simulink model "FFM_Punch"  (R2017a)
settings: Solver=ode3  StartTime=0.0  StopTime=timesteps  FixedStep=data.SIM.Ts  RelTol=1e-3  EnableMultiTasking=on
values from neighbouring files (symbols this model uses):
  data =     [dakota_config.mat]
  downshift_map = data.TCU.upshift.veh_spd_default    [Simulation_results.m]
  upshift_map = data.TCU.upshift.veh_spd_default    [Simulation_results.m]
undefined symbols (not defined in the file or in its folder): air_density, Cd, DiscIntNeverNeededParam, fr_crankshaft, fr_speed_values, g, i_FD, ICE, Low_Ratio, M_Eng_Max, M_Eng_Max_Max, M_Eng_Max_Rpm, mt2m_f, mu_Roll_C0, mu_Roll_C1, mu_Roll_C2, Mv, n_Idle_Eng, Overdrive_Ratio, Re, S_eff_drag, Ts
(part 1 of 15)
settings Model: Creator=37sr  LastModifiedBy=DOM
settings SolverCC: MaxConsecutiveMinStep=Ts
settings DataIOCC: SaveFormat=Array  InspectSignalLogs=on
settings OptimizationCC: LifeSpan=inf
settings DebuggingCC: InheritedTsInSrcMsg=none  ParameterPrecisionLossMsg=none  SFUnexpectedBacktrackingDiag=warning  SFNoUnconditionalDefaultTransitionDiag=warning  SFExecutionAtInitializationDiag=none
settings HardwareCC: ProdBitPerPointer=32  ProdBitPerSizeT=32  ProdBitPerPtrDiffT=32  ProdLargestAtomicFloat=None  ProdIntDivRoundTo=Undefined  ProdEndianess=Unspecified  ProdWordSize=32  ProdHWDeviceType=32-bit Generic
settings ModelReferenceCC: PropagateSignalLabelsOutOfModel=off
settings GRTTargetCC: TargetLangStandard=C89/C90 (ANSI)  GeneratePreprocessorConditionals=Disable all
settings ConfigComp: CovMetricSettings=dw  CovHtmlReporting=on  CovSaveCumulativeToWorkspaceVar=on  CovSaveSingleToWorkspaceVar=on  CovExternalEMLEnable=off
settings ConfigurationSet: Description=SimMechanics 2G

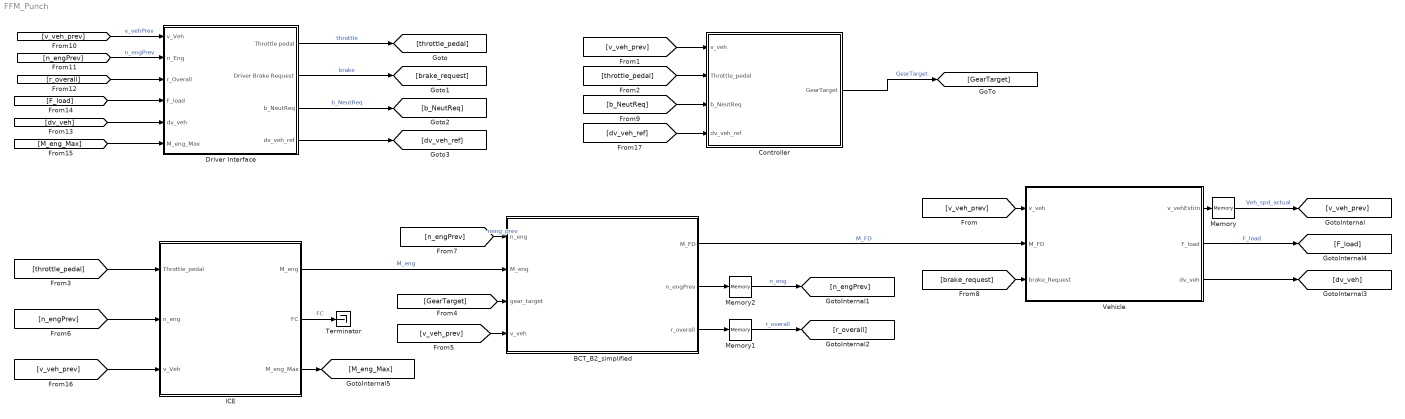
== system FFM_Punch ==
  BCT_B2_simplified : Subsystem
      mask Display:
      | port_label('input',1,'n_eng')
      | port_label('input',2,'M_eng')
      | port_label('input',4,'v_veh')
      | port_label('input',3,'GearTarget')
      | port_label('output',1,'M_FD')
  Controller : Subsystem  Tag=Controls_Lib  Description=SubSystem
      settings: RTWSystemCode=Inline
  Driver Interface : Subsystem
  ICE : Subsystem  SystemSampleTime=Ts/10
      mask Display:
      | port_label('input',1,'Throttle pedal')
      | port_label('input',2,'Engine speed')
      | port_label('output',1,'M_eng')
      | port_label('output',2,'FC')
      | color('blue')
  Memory : Memory  InheritSampleTime=on  LinearizeMemory=on  LinearizeAsDelay=on
  Memory1 : Memory
  Memory2 : Memory  X0=data.ENG.idle_speed
  Terminator : Terminator
      settings: Tag=Controls_Lib  Description=Terminator
  Vehicle : Subsystem  DialogController=PMDialogs.PMDefaultMaskDlg
      mask Display:
      | port_label('input', 1, 'v_veh');
      | port_label('input', 2, 'M_FD');
      | port_label('output', 1, 'v_veh');
  wires:
  Vehicle/1(v_vehEstim) -> Memory/1
  Memory/1 -> [v_veh_prev]  "Veh_spd_actual"
  [v_veh_prev] -> Vehicle/1(v_veh)
  [v_veh_prev] -> Controller/1(v_veh)
  ICE/1(M_eng) -> BCT_B2_simplified/2(M_eng)  "M_eng"
  BCT_B2_simplified/1(M_FD) -> Vehicle/2(M_FD)  "M_FD"
  [throttle_pedal] -> Controller/2(Throttle_pedal)
  [throttle_pedal] -> ICE/1(Throttle_pedal)
  Controller/1(GearTarget) -> [GearTarget]  "GearTarget"
  [v_veh_prev] -> BCT_B2_simplified/4(v_veh)
  BCT_B2_simplified/2(n_engPrev) -> Memory2/1
  [n_engPrev] -> ICE/2(n_eng)
  [n_engPrev] -> BCT_B2_simplified/1(n_eng)  "neng_prev"
  Driver Interface/1(Throttle pedal) -> [throttle_pedal]  "throttle"
  Driver Interface/2(Driver Brake Request) -> [brake_request]  "brake"
  [brake_request] -> Vehicle/3(brake_Request)
  Driver Interface/3(b_NeutReq) -> [b_NeutReq]  "b_NeutReq"
  [b_NeutReq] -> Controller/3(b_NeutReq)
  BCT_B2_simplified/3(r_overall) -> Memory1/1
  ICE/2(FC) -> Terminator/1  "FC"
  [v_veh_prev] -> Driver Interface/1(v_Veh)  "v_vehPrev"
  [n_engPrev] -> Driver Interface/2(n_Eng)  "n_engPrev"
  [r_overall] -> Driver Interface/3(r_Overall)
  Memory2/1 -> [n_engPrev]  "n_eng"
  Memory1/1 -> [r_overall]  "r_overall"
  [GearTarget] -> BCT_B2_simplified/3(gear_target)
  Vehicle/2(F_load) -> [F_load]  "F_load"
  [F_load] -> Driver Interface/4(F_load)
  [v_veh_prev] -> ICE/3(v_Veh)
  Vehicle/3(dv_veh) -> [dv_veh]
  [dv_veh] -> Driver Interface/5(dv_veh)
  ICE/3(M_eng_Max) -> [M_eng_Max]
  [M_eng_Max] -> Driver Interface/6(M_eng_Max)
  Driver Interface/4(dv_veh_ref) -> [dv_veh_ref]
  [dv_veh_ref] -> Controller/4(dv_veh_ref)

== system FFM_Punch/BCT_B2_simplified ==
  n_eng : Inport
  M_eng : Inport  Port=2
  gear_target : Inport  Port=3
  v_veh : Inport  Port=4
  Efficiency_Simplified_Model : Subsystem
  GearBox : Subsystem
      mask Display: image(imread('BCT1_GearCluster.jpg'));
  M_FD : Outport
  n_engPrev : Outport  Port=2
  r_overall : Outport  Port=3
  wires:
  n_eng/1 -> [n_eng]
  M_eng/1 -> [M_inpMeas]
  [M_inpMeas] -> Efficiency_Simplified_Model/2(M_inpMeas)
  [n_eng] -> Efficiency_Simplified_Model/3(n_Eng)
  gear_target/1 -> [gear_target]
  [gear_target] -> Efficiency_Simplified_Model/1(gear_target)
  [gear_target] -> GearBox/1(gear_target)
  Efficiency_Simplified_Model/1(M_inpLoss) -> GearBox/2(M_inpLoss)
  GearBox/1(M_FD) -> M_FD/1
  v_veh/1 -> [v_veh]
  GearBox/2(n_engPrev) -> n_engPrev/1
  [v_veh] -> GearBox/3(v_veh)
  GearBox/3(r_overall) -> r_overall/1

== system FFM_Punch/Controller ==
  v_veh : Inport  Tag=Controls_Lib  Description=Inp  Interpolate=off
  Throttle_pedal : Inport  Port=2
  b_NeutReq : Inport  Port=3
  dv_veh_ref : Inport  Tag=Controls_Lib  Description=Inp  Port=4  Interpolate=off
  F02_03_03_03_Shift_Laws_Determination : Subsystem
  F02_03_03_05_Raw_Gear_Target_Auto_Mode : Subsystem
  Scope : Scope  NumInputPorts=2
  Scope1 : Scope
  Scope2 : Scope
  UnitDelay : UnitDelay  Tag=Controls_Lib  Description=UnitDelay  InitialCondition=X0  SampleTime=SampleTime  mask(Unit delay){X0=0, InputProcessing=Elements as channels (sample based), SampleTime=-1, StateIdentifier=, StateMustResolveToSignalObject=off, RTWStateStorageClass=Auto, RTWStateStorageTypeQualifier=}
      mask prompts: X0 "Initial conditions:"; InputProcessing "Input processing:"; SampleTime "Sample time (-1 for inherited):"; StateIdentifier "State name:"; StateMustResolveToSignalObject "State name must resolve to Simulink signal object"; RTWStateStorageClass "Code generation storage class:"; RTWStateStorageTypeQualifier "Code generation storage type qualifier:"
      mask help: Delays input signal by one sample period
      settings: AttributesFormatString=Init_con=%<X0>
      mask Help: web([fileparts(which('Lib_discrete')) filesep 'hlp' filesep 'lib_UnitDelay.html'], '-helpbrowser')
      mask TypeOptions X0: X0
      mask TypeOptions InputProcessing: InputProcessing
      mask TypeOptions SampleTime: SampleTime
      mask TypeOptions StateIdentifier: StateIdentifier
      mask TypeOptions StateMustResolveToSignalObject: StateMustResolveToSignalObject
      mask TypeOptions RTWStateStorageClass: RTWStateStorageClass
      mask TypeOptions RTWStateStorageTypeQualifier: RTWStateStorageTypeQualifier
  GearTarget : Outport  Tag=Controls_Lib  Description=Out  InitialOutput=0
  wires:
  Throttle_pedal/1 -> F02_03_03_03_Shift_Laws_Determination/1(Throttle_pedal)
  F02_03_03_03_Shift_Laws_Determination/1(ts_v_vectThdAutoModDown) -> Scope1/1, [ts_v_vectThdAutoModDown]
  F02_03_03_03_Shift_Laws_Determination/2(ts_v_vectThdAutoModUp) -> Scope2/1, [ts_v_vectThdAutoModUp]
  [ts_v_vectThdAutoModDown] -> F02_03_03_05_Raw_Gear_Target_Auto_Mode/1(ts_v_vectThdAutoModDown)
  [ts_v_vectThdAutoModUp] -> F02_03_03_05_Raw_Gear_Target_Auto_Mode/2(ts_v_vectThdAutoModUp)
  [ts_z_gearTgtFwd] -> F02_03_03_05_Raw_Gear_Target_Auto_Mode/3(ts_z_gearTgtFwd)
  v_veh/1 -> Scope/2, F02_03_03_05_Raw_Gear_Target_Auto_Mode/4(vehest_v_frntWhl)
  F02_03_03_05_Raw_Gear_Target_Auto_Mode/1(ts_z_autoGearTgtRaw) -> UnitDelay/1, GearTarget/1
  UnitDelay/1 -> [ts_z_gearTgtFwd]
  b_NeutReq/1 -> F02_03_03_05_Raw_Gear_Target_Auto_Mode/5(b_NeutReq)
  [dv_veh_ref] -> F02_03_03_05_Raw_Gear_Target_Auto_Mode/6(dv_veh_ref)
  dv_veh_ref/1 -> Scope/1, [dv_veh_ref]

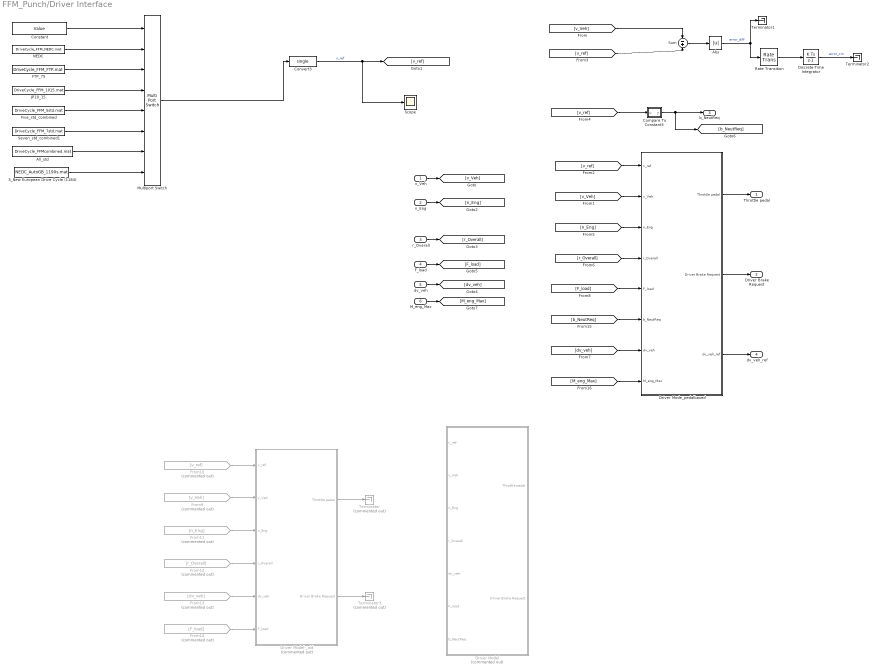
== system FFM_Punch/Driver Interface ==
  v_Veh : Inport
  n_Eng : Inport  Port=2
  r_Overall : Inport  Port=3
  F_load : Inport  Port=4
  dv_veh : Inport  Port=5
  M_eng_Max : Inport  Port=6
  3_New European Drive Cycle (1184) : FromFile  FileName=NEDC_AutoGB_1190s.mat  SampleTime=data.SIM.Ts
  Abs : Abs
  All_std : FromFile  FileName=DriveCycle_FFMcombined.mat  SampleTime=0
  Compare To Constant3 : Subsystem  mask(Compare To Constant){relop=<, const=0.5, OutDataTypeStr=boolean, ZeroCross=off}
      mask prompts: relop "Simulink:masks:Operator_MP"; const "Simulink:masks:ConstantValue_MP"; OutDataTypeStr "Simulink:masks:OutputDataType_MP"; ZeroCross "Simulink:masks:EnableZerocrossingDetection_MP"
      mask help: Simulink:masks:CompareToConstant_MD
      mask init:
      | blkName = gcb;
      | 
      | if strcmp(get_param(gcbh,'OutDataTypeStr'),'boolean')
      | 	setValue = 'boolean';
      | else
      | 	setValue = 'fixdt(0, 8)';
      | end
      | 
      | set_param([blkName,'/Compare'],'relop',relop, ...
      | 	'OutDataTypeStr', setValue, 'ZeroCross', ZeroCross);
      | 
      | str = [relop,' C']; %default
      | 
      | const_str = get_param(blkName, 'const');
      | const_val = str2num(const_str);
      | 
      | if isempty(const_val) %#ok<ST2NM>
      |     %Expression/Variable
      |     str = [relop, ' ', strtrim(const_str)];
      | else
      |     if length(const_val) == 1 
      |         if Simulink.data.isSupportedEnumClass(class(const_val))
      |             % Special Handling for Enumerations
      |             if Simulink.data.getEnumTypeInfo(class(const_val), 'AddClassNameToEnumNames')
      |                 str = [relop, ' ', strtrim(const_str)];
      |             else
      |                 str = [relop, ' ', char(const_val)];
      |             end
      |         elseif(isfloat(const_val) || isinteger(const_val)) 
      |                 str = [relop, ' ', num2str(const_val)];
      |         end
      |     end
      | end
      mask TypeOptions relop: == | ~= | < | <= | >= | >
      mask TypeOptions OutDataTypeStr: Simulink:masks:uint8 | Simulink:masks:boolean
      mask Callback ZeroCross: sl('zeroCrossEnable', gcbh);
      mask Display: disp(str)
  Constant : Constant  Tag=Controls_Lib  Description=constant  Value=Value  OutMin=OutMin  OutMax=OutMax  OutDataTypeStr=Inherit: Inherit via back propagation  SampleTime=SampleTime  FramePeriod=FramePeriod  mask(Constant){Value=data.SIM.drivecycle, VectorParams1D=on, SampleTime=-1, FramePeriod=inf, OutMin=[], OutMax=[], OutDataTypeStr=Inherit: Inherit via back propagation, LockScale=off}
      mask prompts: Value "Simulink:blkprm_prompts:ConstConstValue"; VectorParams1D "Simulink:blkprm_prompts:AllSrcsVector1D"; SampleTime "Simulink:blkprm_prompts:AllSrcBlksSampleTime"; FramePeriod "Simulink:blkprm_prompts:AllSrcBlksFramePeriod"; OutMin "Simulink:blkprm_prompts:OutputDesignMin"; OutMax "Simulink:blkprm_prompts:OutputDesignMax"; OutDataTypeStr "Simulink:blkprm_prompts:OUTPUT_UNIFIEDDATATYPE"; LockScale "Simulink:blkprm_prompts:LockScale"
      mask help: Output the constant specified by the 'Constant value' parameter.
      mask Help: web([fileparts(which('Lib_built')) filesep 'hlp' filesep 'lib_constant' '.html'], '-helpbrowser')
      mask TypeOptions Value: Value
      mask TypeOptions VectorParams1D: VectorParams1D
      mask TypeOptions SampleTime: SampleTime
      mask TypeOptions FramePeriod: FramePeriod
      mask TypeOptions OutMin: OutMin
      mask TypeOptions OutMax: OutMax
      mask TypeOptions OutDataTypeStr: OutDataTypeStr
      mask TypeOptions LockScale: LockScale
      mask DialogControl ParameterTabVar0 Prompt: Main
      mask Display: disp(get_param(gcb,'Value'))
  Convert3 : DataTypeConversion  Tag=Controls_Lib  Description=Convert  OutMin=OutMin  OutMax=OutMax  OutDataTypeStr=single  RndMeth=Round  SampleTime=SampleTime  SaturateOnIntegerOverflow=on  mask(Datatype conversion){ConvertRealWorld=Real World Value (RWV), SampleTime=-1, OutMin=[], OutMax=[], OutDataTypeStr=single, LockScale=off, RndMeth=Round, SaturateOnIntegerOverflow=on}
      mask prompts: ConvertRealWorld "Input and output to have equal:"; SampleTime "Sample time (-1 for inherited):"; OutMin "Output minimum:"; OutMax "Output maximum:"; OutDataTypeStr "Output data type:"; LockScale "Lock output data type setting against changes by the fixed-point tools"; RndMeth "Integer rounding mode:"; SaturateOnIntegerOverflow "Saturate on integer overflow"
      mask help: Convert the input to the data type and scaling of the output.
      mask Help: web([fileparts(which('Lib_built')) filesep 'hlp' filesep 'lib_DataTypeConv' '.html'], '-helpbrowser')
      mask TypeOptions ConvertRealWorld: ConvertRealWorld
      mask TypeOptions SampleTime: SampleTime
      mask TypeOptions OutMin: OutMin
      mask TypeOptions OutMax: OutMax
      mask TypeOptions OutDataTypeStr: OutDataTypeStr
      mask TypeOptions LockScale: LockScale
      mask TypeOptions RndMeth: RndMeth
      mask TypeOptions SaturateOnIntegerOverflow: SaturateOnIntegerOverflow
  Discrete-Time Integrator : DiscreteIntegrator  InitialConditionSetting=State (most efficient)  OutDataTypeStr=Inherit: Inherit via back propagation  ICPrevOutput=DiscIntNeverNeededParam  ICPrevScaledInput=DiscIntNeverNeededParam
  Driver Mode_pedalbased : Subsystem
  Driver Model : Subsystem  Commented=on
  Driver Model-_old : Subsystem  Commented=on
  FTP_75 : FromFile  FileName=DriveCycle_FFM_FTP.mat  SampleTime=0
  Five_std_combined : FromFile  FileName=DriveCycle_FFM_5std.mat  SampleTime=0
  From10 : From  Tag=Controls_Lib  Description=FromInternal  Commented=on  GotoTag=v_ref
  From11 : From  Tag=Controls_Lib  Description=FromInternal  Commented=on  GotoTag=n_Eng
  From12 : From  Tag=Controls_Lib  Description=FromInternal  Commented=on  GotoTag=r_Overall
  From13 : From  Tag=Controls_Lib  Description=FromInternal  Commented=on  GotoTag=dv_veh
  From14 : From  Tag=Controls_Lib  Description=FromInternal  Commented=on  GotoTag=F_load
  From9 : From  Tag=Controls_Lib  Description=FromInternal  Commented=on  GotoTag=v_Veh
  JP10_15 : FromFile  FileName=DriveCycle_FFM_1015.mat  SampleTime=0
  Multiport Switch : MultiPortSwitch  Inputs=6  DataPortForDefault=Additional data port
  NEDC : FromFile  FileName=DriveCycle_FFM_NEDC.mat  SampleTime=0
  Rate Transition : RateTransition
  Scope : Scope
  Seven_std_combined1 : FromFile  FileName=DriveCycle_FFM_7std.mat  SampleTime=0
  Sum : Sum  Inputs=-+
  Terminator : Terminator  Commented=on
  Terminator1 : Terminator
  Terminator2 : Terminator
  Terminator3 : Terminator  Commented=on
  Throttle pedal : Outport
  Driver Brake Request : Outport  Port=2
  b_NeutReq : Outport  Port=3
  dv_veh_ref : Outport  Port=4
  wires:
  Sum/1 -> Abs/1
  Abs/1 -> Terminator1/1, Rate Transition/1  "error_diff"
  Discrete-Time Integrator/1 -> Terminator2/1  "error_cm"
  Rate Transition/1 -> Discrete-Time Integrator/1
  v_Veh/1 -> [v_Veh]
  [v_Veh] -> Sum/1
  3_New European Drive Cycle (1184)/1 -> Multiport Switch/8
  Convert3/1 -> Scope/1, [v_ref]  "v_ref"
  Constant/1 -> Multiport Switch/1
  [v_ref] -> Sum/2
  [v_ref] -> Compare To Constant3/1(u)
  Compare To Constant3/1(y) -> [b_NeutReq], b_NeutReq/1
  n_Eng/1 -> [n_Eng]
  r_Overall/1 -> [r_Overall]
  F_load/1 -> [F_load]
  From10/1 -> Driver Model-_old/1(v_ref)
  From14/1 -> Driver Model-_old/6(F_load)
  From12/1 -> Driver Model-_old/4(r_Overall)
  From11/1 -> Driver Model-_old/3(n_Eng)
  From13/1 -> Driver Model-_old/5(dv_veh)
  From9/1 -> Driver Model-_old/2(v_Veh)
  Driver Model-_old/1(Throttle pedal) -> Terminator/1
  Driver Model-_old/2(Driver Brake Request) -> Terminator3/1
  [v_ref] -> Driver Mode_pedalbased/1(v_ref)
  [v_Veh] -> Driver Mode_pedalbased/2(v_Veh)
  [n_Eng] -> Driver Mode_pedalbased/3(n_Eng)
  [r_Overall] -> Driver Mode_pedalbased/4(r_Overall)
  [F_load] -> Driver Mode_pedalbased/5(F_load)
  [b_NeutReq] -> Driver Mode_pedalbased/6(b_NeutReq)
  Driver Mode_pedalbased/1(Throttle pedal) -> Throttle pedal/1
  Driver Mode_pedalbased/2(Driver Brake Request) -> Driver Brake Request/1
  dv_veh/1 -> [dv_veh]
  [dv_veh] -> Driver Mode_pedalbased/7(dv_veh)
  Multiport Switch/1 -> Convert3/1
  M_eng_Max/1 -> [M_eng_Max]
  [M_eng_Max] -> Driver Mode_pedalbased/8(M_eng_Max)
  Driver Mode_pedalbased/3(dv_veh_ref) -> dv_veh_ref/1
  All_std/1 -> Multiport Switch/7
  FTP_75/1 -> Multiport Switch/3
  NEDC/1 -> Multiport Switch/2
  JP10_15/1 -> Multiport Switch/4
  Five_std_combined/1 -> Multiport Switch/5
  Seven_std_combined1/1 -> Multiport Switch/6

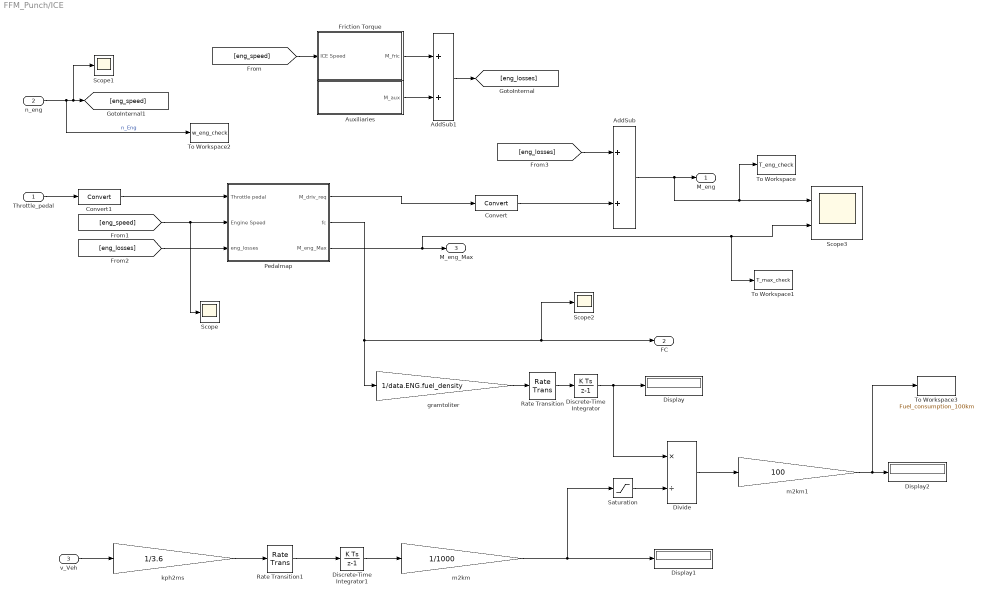
== system FFM_Punch/ICE ==
  Throttle_pedal : Inport
  n_eng : Inport  Port=2
  v_Veh : Inport  Port=3
  AddSub : Sum  Tag=Controls_Lib  Description=AddSub  CollapseDim=CollapseDim  AccumDataTypeStr=single  OutMin=OutMin  OutMax=OutMax  OutDataTypeStr=single  RndMeth=Nearest  SampleTime=SampleTime  InputSameDT=on  mask(AddSub){IconShape=rectangular, Inputs=++, CollapseMode=All dimensions, CollapseDim=1, SampleTime=-1, InputSameDT=on, AccumDataTypeStr=single, OutMin=[], OutMax=[], OutDataTypeStr=single, LockScale=off, RndMeth=Nearest, SaturateOnIntegerOverflow=off}
      mask prompts: IconShape "Icon shape:"; Inputs "List of signs:"; CollapseMode "Sum over:"; CollapseDim "Dimension:"; SampleTime "Sample time (-1 for inherited):"; InputSameDT "Require all inputs to have the same data type"; AccumDataTypeStr "Accumulator data type:"; OutMin "Output minimum:"; OutMax "Output maximum:"; OutDataTypeStr "Output data type:"; LockScale "Lock data type settings against changes by the fixed-point tools"; RndMeth "Integer rounding mode:"; SaturateOnIntegerOverflow "Saturate on integer overflow"
      mask help:
      | Add or subtract inputs.  Specify one of the following:
      | a) string containing + or - for each input port, | for spacer between ports (e.g. ++|-|++)
      | b) scalar, >= 1, specifies the number of input ports to be summed.
      | When there is only one input port, add or subtract elements over all dimensions or one specified dimension
      mask Help: web([fileparts(which('Lib_built')) filesep 'hlp' filesep 'lib_AddSub' '.html'], '-helpbrowser')
      mask TypeOptions IconShape: IconShape
      mask TypeOptions Inputs: Inputs
      mask TypeOptions CollapseMode: CollapseMode
      mask TypeOptions CollapseDim: CollapseDim
      mask TypeOptions SampleTime: SampleTime
      mask TypeOptions InputSameDT: InputSameDT
      mask TypeOptions AccumDataTypeStr: AccumDataTypeStr
      mask TypeOptions OutMin: OutMin
      mask TypeOptions OutMax: OutMax
      mask TypeOptions OutDataTypeStr: OutDataTypeStr
      mask TypeOptions LockScale: LockScale
      mask TypeOptions RndMeth: RndMeth
      mask TypeOptions SaturateOnIntegerOverflow: SaturateOnIntegerOverflow
  AddSub1 : Sum  Tag=Controls_Lib  Description=AddSub  CollapseDim=CollapseDim  AccumDataTypeStr=single  OutMin=OutMin  OutMax=OutMax  OutDataTypeStr=single  RndMeth=Nearest  SampleTime=SampleTime  InputSameDT=on  mask(AddSub){IconShape=rectangular, Inputs=++, CollapseMode=All dimensions, CollapseDim=1, SampleTime=-1, InputSameDT=on, AccumDataTypeStr=single, OutMin=[], OutMax=[], OutDataTypeStr=single, LockScale=off, RndMeth=Nearest, SaturateOnIntegerOverflow=off}
      mask prompts: IconShape "Icon shape:"; Inputs "List of signs:"; CollapseMode "Sum over:"; CollapseDim "Dimension:"; SampleTime "Sample time (-1 for inherited):"; InputSameDT "Require all inputs to have the same data type"; AccumDataTypeStr "Accumulator data type:"; OutMin "Output minimum:"; OutMax "Output maximum:"; OutDataTypeStr "Output data type:"; LockScale "Lock data type settings against changes by the fixed-point tools"; RndMeth "Integer rounding mode:"; SaturateOnIntegerOverflow "Saturate on integer overflow"
      mask help:
      | Add or subtract inputs.  Specify one of the following:
      | a) string containing + or - for each input port, | for spacer between ports (e.g. ++|-|++)
      | b) scalar, >= 1, specifies the number of input ports to be summed.
      | When there is only one input port, add or subtract elements over all dimensions or one specified dimension
      mask Help: web([fileparts(which('Lib_built')) filesep 'hlp' filesep 'lib_AddSub' '.html'], '-helpbrowser')
      mask TypeOptions IconShape: IconShape
      mask TypeOptions Inputs: Inputs
      mask TypeOptions CollapseMode: CollapseMode
      mask TypeOptions CollapseDim: CollapseDim
      mask TypeOptions SampleTime: SampleTime
      mask TypeOptions InputSameDT: InputSameDT
      mask TypeOptions AccumDataTypeStr: AccumDataTypeStr
      mask TypeOptions OutMin: OutMin
      mask TypeOptions OutMax: OutMax
      mask TypeOptions OutDataTypeStr: OutDataTypeStr
      mask TypeOptions LockScale: LockScale
      mask TypeOptions RndMeth: RndMeth
      mask TypeOptions SaturateOnIntegerOverflow: SaturateOnIntegerOverflow
  Auxiliaries : Subsystem
  Convert : DataTypeConversion  Tag=Controls_Lib  Description=Convert  OutMin=OutMin  OutMax=OutMax  RndMeth=Round  SampleTime=SampleTime  SaturateOnIntegerOverflow=on  mask(Datatype conversion){ConvertRealWorld=Real World Value (RWV), SampleTime=-1, OutMin=[], OutMax=[], OutDataTypeStr=Inherit: Inherit via back propagation, LockScale=off, RndMeth=Round, SaturateOnIntegerOverflow=on}
      mask prompts: ConvertRealWorld "Input and output to have equal:"; SampleTime "Sample time (-1 for inherited):"; OutMin "Output minimum:"; OutMax "Output maximum:"; OutDataTypeStr "Output data type:"; LockScale "Lock output data type setting against changes by the fixed-point tools"; RndMeth "Integer rounding mode:"; SaturateOnIntegerOverflow "Saturate on integer overflow"
      mask help: Convert the input to the data type and scaling of the output.
      mask Help: web([fileparts(which('Lib_built')) filesep 'hlp' filesep 'lib_DataTypeConv' '.html'], '-helpbrowser')
      mask TypeOptions ConvertRealWorld: ConvertRealWorld
      mask TypeOptions SampleTime: SampleTime
      mask TypeOptions OutMin: OutMin
      mask TypeOptions OutMax: OutMax
      mask TypeOptions OutDataTypeStr: OutDataTypeStr
      mask TypeOptions LockScale: LockScale
      mask TypeOptions RndMeth: RndMeth
      mask TypeOptions SaturateOnIntegerOverflow: SaturateOnIntegerOverflow
  Convert1 : DataTypeConversion  Tag=Controls_Lib  Description=Convert  OutMin=OutMin  OutMax=OutMax  RndMeth=Round  SampleTime=SampleTime  SaturateOnIntegerOverflow=on  mask(Datatype conversion){ConvertRealWorld=Real World Value (RWV), SampleTime=-1, OutMin=[], OutMax=[], OutDataTypeStr=Inherit: Inherit via back propagation, LockScale=off, RndMeth=Round, SaturateOnIntegerOverflow=on}
      mask prompts: ConvertRealWorld "Input and output to have equal:"; SampleTime "Sample time (-1 for inherited):"; OutMin "Output minimum:"; OutMax "Output maximum:"; OutDataTypeStr "Output data type:"; LockScale "Lock output data type setting against changes by the fixed-point tools"; RndMeth "Integer rounding mode:"; SaturateOnIntegerOverflow "Saturate on integer overflow"
      mask help: Convert the input to the data type and scaling of the output.
      mask Help: web([fileparts(which('Lib_built')) filesep 'hlp' filesep 'lib_DataTypeConv' '.html'], '-helpbrowser')
      mask TypeOptions ConvertRealWorld: ConvertRealWorld
      mask TypeOptions SampleTime: SampleTime
      mask TypeOptions OutMin: OutMin
      mask TypeOptions OutMax: OutMax
      mask TypeOptions OutDataTypeStr: OutDataTypeStr
      mask TypeOptions LockScale: LockScale
      mask TypeOptions RndMeth: RndMeth
      mask TypeOptions SaturateOnIntegerOverflow: SaturateOnIntegerOverflow
  Discrete-Time Integrator : DiscreteIntegrator  InitialConditionSetting=State (most efficient)  ICPrevOutput=DiscIntNeverNeededParam  ICPrevScaledInput=DiscIntNeverNeededParam
  Discrete-Time Integrator1 : DiscreteIntegrator  InitialConditionSetting=State (most efficient)  ICPrevOutput=DiscIntNeverNeededParam  ICPrevScaledInput=DiscIntNeverNeededParam
  Display : Display
  Display1 : Display
  Display2 : Display
  Divide : Product  Inputs=*/
  Friction Torque : Subsystem
  Pedalmap : Subsystem
  Rate Transition : RateTransition
  Rate Transition1 : RateTransition
  Saturation : Saturate  UpperLimit=100000  LowerLimit=data.SIM.eps
  Scope : Scope
  Scope1 : Scope
  Scope2 : Scope
  Scope3 : Scope  NumInputPorts=2
  To Workspace : ToWorkspace  VariableName=T_eng_check  SampleTime=-1
  To Workspace1 : ToWorkspace  VariableName=T_max_check  SampleTime=-1
  To Workspace2 : ToWorkspace  VariableName=w_eng_check  SampleTime=-1
  To Workspace3 : ToWorkspace  VariableName=Fuel_consumption_100km  SampleTime=-1
  gramtoliter : Gain  Gain=1/data.ENG.fuel_density
  kph2ms : Gain  Gain=1/3.6
  m2km : Gain  Gain=1/1000
  m2km1 : Gain  Gain=100
  M_eng : Outport
  FC : Outport  Port=2
  M_eng_Max : Outport  Port=3
  wires:
  [eng_speed] -> Friction Torque/1(ICE Speed)
  Auxiliaries/1(M_aux) -> AddSub1/2
  Friction Torque/1(M_fric) -> AddSub1/1
  AddSub/1 -> To Workspace/1, Scope3/1, M_eng/1
  Pedalmap/1(M_driv_req) -> Convert/1
  Pedalmap/2(fc) -> Scope2/1, FC/1, gramtoliter/1
  Throttle_pedal/1 -> Convert1/1
  n_eng/1 -> To Workspace2/1, Scope1/1, [eng_speed]  "n_Eng"
  [eng_speed] -> Scope/1, Pedalmap/2(Engine Speed)
  AddSub1/1 -> [eng_losses]
  [eng_losses] -> AddSub/1
  [eng_losses] -> Pedalmap/3(eng_losses)
  Convert/1 -> AddSub/2
  Convert1/1 -> Pedalmap/1("Throttle pedal  ")
  Discrete-Time Integrator/1 -> Divide/1, Display/1
  Rate Transition/1 -> Discrete-Time Integrator/1
  gramtoliter/1 -> Rate Transition/1
  v_Veh/1 -> kph2ms/1
  Rate Transition1/1 -> Discrete-Time Integrator1/1
  Discrete-Time Integrator1/1 -> m2km/1
  kph2ms/1 -> Rate Transition1/1
  m2km/1 -> Saturation/1, Display1/1
  Divide/1 -> m2km1/1
  m2km1/1 -> To Workspace3/1, Display2/1
  Saturation/1 -> Divide/2
  Pedalmap/3(M_eng_Max) -> To Workspace1/1, Scope3/2, M_eng_Max/1

== system FFM_Punch/Vehicle ==
  v_veh : Inport  Tag=Controls_Lib  Description=Inp  Interpolate=off
  M_FD : Inport  Tag=Controls_Lib  Description=Inp  Port=2  Interpolate=off
  brake_Request : Inport  Port=3
  Abs : Abs  RndMeth=Zero  SaturateOnIntegerOverflow=on
  AddSub : Sum  Tag=Controls_Lib  Description=AddSub  CollapseDim=CollapseDim  AccumDataTypeStr=single  OutMin=OutMin  OutMax=OutMax  OutDataTypeStr=single  RndMeth=Nearest  SampleTime=SampleTime  InputSameDT=on  mask(AddSub){IconShape=rectangular, Inputs=++, CollapseMode=All dimensions, CollapseDim=1, SampleTime=-1, InputSameDT=on, AccumDataTypeStr=single, OutMin=[], OutMax=[], OutDataTypeStr=single, LockScale=off, RndMeth=Nearest, SaturateOnIntegerOverflow=off}
      mask prompts: IconShape "Icon shape:"; Inputs "List of signs:"; CollapseMode "Sum over:"; CollapseDim "Dimension:"; SampleTime "Sample time (-1 for inherited):"; InputSameDT "Require all inputs to have the same data type"; AccumDataTypeStr "Accumulator data type:"; OutMin "Output minimum:"; OutMax "Output maximum:"; OutDataTypeStr "Output data type:"; LockScale "Lock data type settings against changes by the fixed-point tools"; RndMeth "Integer rounding mode:"; SaturateOnIntegerOverflow "Saturate on integer overflow"
      mask help:
      | Add or subtract inputs.  Specify one of the following:
      | a) string containing + or - for each input port, | for spacer between ports (e.g. ++|-|++)
      | b) scalar, >= 1, specifies the number of input ports to be summed.
      | When there is only one input port, add or subtract elements over all dimensions or one specified dimension
      mask Help: web([fileparts(which('Lib_built')) filesep 'hlp' filesep 'lib_AddSub' '.html'], '-helpbrowser')
      mask TypeOptions IconShape: IconShape
      mask TypeOptions Inputs: Inputs
      mask TypeOptions CollapseMode: CollapseMode
      mask TypeOptions CollapseDim: CollapseDim
      mask TypeOptions SampleTime: SampleTime
      mask TypeOptions InputSameDT: InputSameDT
      mask TypeOptions AccumDataTypeStr: AccumDataTypeStr
      mask TypeOptions OutMin: OutMin
      mask TypeOptions OutMax: OutMax
      mask TypeOptions OutDataTypeStr: OutDataTypeStr
      mask TypeOptions LockScale: LockScale
      mask TypeOptions RndMeth: RndMeth
      mask TypeOptions SaturateOnIntegerOverflow: SaturateOnIntegerOverflow
  AddSub1 : Sum  Tag=Controls_Lib  Description=AddSub  Inputs=-+  CollapseDim=CollapseDim  AccumDataTypeStr=single  OutMin=OutMin  OutMax=OutMax  OutDataTypeStr=single  RndMeth=Nearest  SampleTime=SampleTime  InputSameDT=on  mask(AddSub){IconShape=rectangular, Inputs=-+, CollapseMode=All dimensions, CollapseDim=1, SampleTime=-1, InputSameDT=on, AccumDataTypeStr=single, OutMin=[], OutMax=[], OutDataTypeStr=single, LockScale=off, RndMeth=Nearest, SaturateOnIntegerOverflow=off}
      mask prompts: IconShape "Icon shape:"; Inputs "List of signs:"; CollapseMode "Sum over:"; CollapseDim "Dimension:"; SampleTime "Sample time (-1 for inherited):"; InputSameDT "Require all inputs to have the same data type"; AccumDataTypeStr "Accumulator data type:"; OutMin "Output minimum:"; OutMax "Output maximum:"; OutDataTypeStr "Output data type:"; LockScale "Lock data type settings against changes by the fixed-point tools"; RndMeth "Integer rounding mode:"; SaturateOnIntegerOverflow "Saturate on integer overflow"
      mask help:
      | Add or subtract inputs.  Specify one of the following:
      | a) string containing + or - for each input port, | for spacer between ports (e.g. ++|-|++)
      | b) scalar, >= 1, specifies the number of input ports to be summed.
      | When there is only one input port, add or subtract elements over all dimensions or one specified dimension
      mask Help: web([fileparts(which('Lib_built')) filesep 'hlp' filesep 'lib_AddSub' '.html'], '-helpbrowser')
      mask TypeOptions IconShape: IconShape
      mask TypeOptions Inputs: Inputs
      mask TypeOptions CollapseMode: CollapseMode
      mask TypeOptions CollapseDim: CollapseDim
      mask TypeOptions SampleTime: SampleTime
      mask TypeOptions InputSameDT: InputSameDT
      mask TypeOptions AccumDataTypeStr: AccumDataTypeStr
      mask TypeOptions OutMin: OutMin
      mask TypeOptions OutMax: OutMax
      mask TypeOptions OutDataTypeStr: OutDataTypeStr
      mask TypeOptions LockScale: LockScale
      mask TypeOptions RndMeth: RndMeth
      mask TypeOptions SaturateOnIntegerOverflow: SaturateOnIntegerOverflow
  Constant3 : Constant  Tag=Controls_Lib  Description=constant  Value=Value  OutMin=OutMin  OutMax=OutMax  OutDataTypeStr=Inherit: Inherit via back propagation  SampleTime=SampleTime  FramePeriod=FramePeriod  mask(Constant){Value=0.2, VectorParams1D=on, SampleTime=-1, FramePeriod=inf, OutMin=[], OutMax=[], OutDataTypeStr=Inherit: Inherit via back propagation, LockScale=off}
      mask prompts: Value "Simulink:blkprm_prompts:ConstConstValue"; VectorParams1D "Simulink:blkprm_prompts:AllSrcsVector1D"; SampleTime "Simulink:blkprm_prompts:AllSrcBlksSampleTime"; FramePeriod "Simulink:blkprm_prompts:AllSrcBlksFramePeriod"; OutMin "Simulink:blkprm_prompts:OutputDesignMin"; OutMax "Simulink:blkprm_prompts:OutputDesignMax"; OutDataTypeStr "Simulink:blkprm_prompts:OUTPUT_UNIFIEDDATATYPE"; LockScale "Simulink:blkprm_prompts:LockScale"
      mask help: Output the constant specified by the 'Constant value' parameter.
      mask Help: web([fileparts(which('Lib_built')) filesep 'hlp' filesep 'lib_constant' '.html'], '-helpbrowser')
      mask TypeOptions Value: Value
      mask TypeOptions VectorParams1D: VectorParams1D
      mask TypeOptions SampleTime: SampleTime
      mask TypeOptions FramePeriod: FramePeriod
      mask TypeOptions OutMin: OutMin
      mask TypeOptions OutMax: OutMax
      mask TypeOptions OutDataTypeStr: OutDataTypeStr
      mask TypeOptions LockScale: LockScale
      mask DialogControl ParameterTabVar0 Prompt: Main
      mask Display: disp(get_param(gcb,'Value'))
  Constant4 : Constant  Tag=Controls_Lib  Description=constant  Value=Value  OutMin=OutMin  OutMax=OutMax  OutDataTypeStr=Inherit: Inherit via back propagation  SampleTime=SampleTime  FramePeriod=FramePeriod  mask(Constant){Value=0, VectorParams1D=on, SampleTime=-1, FramePeriod=inf, OutMin=[], OutMax=[], OutDataTypeStr=Inherit: Inherit via back propagation, LockScale=off}
      mask prompts: Value "Simulink:blkprm_prompts:ConstConstValue"; VectorParams1D "Simulink:blkprm_prompts:AllSrcsVector1D"; SampleTime "Simulink:blkprm_prompts:AllSrcBlksSampleTime"; FramePeriod "Simulink:blkprm_prompts:AllSrcBlksFramePeriod"; OutMin "Simulink:blkprm_prompts:OutputDesignMin"; OutMax "Simulink:blkprm_prompts:OutputDesignMax"; OutDataTypeStr "Simulink:blkprm_prompts:OUTPUT_UNIFIEDDATATYPE"; LockScale "Simulink:blkprm_prompts:LockScale"
      mask help: Output the constant specified by the 'Constant value' parameter.
      mask Help: web([fileparts(which('Lib_built')) filesep 'hlp' filesep 'lib_constant' '.html'], '-helpbrowser')
      mask TypeOptions Value: Value
      mask TypeOptions VectorParams1D: VectorParams1D
      mask TypeOptions SampleTime: SampleTime
      mask TypeOptions FramePeriod: FramePeriod
      mask TypeOptions OutMin: OutMin
      mask TypeOptions OutMax: OutMax
      mask TypeOptions OutDataTypeStr: OutDataTypeStr
      mask TypeOptions LockScale: LockScale
      mask DialogControl ParameterTabVar0 Prompt: Main
      mask Display: disp(get_param(gcb,'Value'))
  Constant5 : Constant  Tag=Controls_Lib  Description=constant  Value=Value  OutMin=OutMin  OutMax=OutMax  OutDataTypeStr=Inherit: Inherit via back propagation  SampleTime=SampleTime  FramePeriod=FramePeriod  mask(Constant){Value=0, VectorParams1D=on, SampleTime=-1, FramePeriod=inf, OutMin=[], OutMax=[], OutDataTypeStr=Inherit: Inherit via back propagation, LockScale=off}
      mask prompts: Value "Simulink:blkprm_prompts:ConstConstValue"; VectorParams1D "Simulink:blkprm_prompts:AllSrcsVector1D"; SampleTime "Simulink:blkprm_prompts:AllSrcBlksSampleTime"; FramePeriod "Simulink:blkprm_prompts:AllSrcBlksFramePeriod"; OutMin "Simulink:blkprm_prompts:OutputDesignMin"; OutMax "Simulink:blkprm_prompts:OutputDesignMax"; OutDataTypeStr "Simulink:blkprm_prompts:OUTPUT_UNIFIEDDATATYPE"; LockScale "Simulink:blkprm_prompts:LockScale"
      mask help: Output the constant specified by the 'Constant value' parameter.
      mask Help: web([fileparts(which('Lib_built')) filesep 'hlp' filesep 'lib_constant' '.html'], '-helpbrowser')
      mask TypeOptions Value: Value
      mask TypeOptions VectorParams1D: VectorParams1D
      mask TypeOptions SampleTime: SampleTime
      mask TypeOptions FramePeriod: FramePeriod
      mask TypeOptions OutMin: OutMin
      mask TypeOptions OutMax: OutMax
      mask TypeOptions OutDataTypeStr: OutDataTypeStr
      mask TypeOptions LockScale: LockScale
      mask DialogControl ParameterTabVar0 Prompt: Main
      mask Display: disp(get_param(gcb,'Value'))
  Discrete-Time Integrator : DiscreteIntegrator  InitialConditionSetting=State (most efficient)  SampleTime=data.SIM.Ts  ICPrevOutput=DiscIntNeverNeededParam  ICPrevScaledInput=DiscIntNeverNeededParam
  FirstOrderDerivative1 : Subsystem  Tag=Controls_Lib  Description=DiscreteDerivative  mask(Discrete Derivative Block){}
      mask help:
      | Computes the discrete derivative of the input signal as the rate of change of signal with respect to Sampling Time.
      |
      | Inputs:
      | Input         : Signal to be Filtered
      |
      |
      |
      | Outputs:
      | Output : Filter Output of the Discrete Derivative block
      mask Help: web([fileparts(which('Lib_discrete')) filesep 'hlp' filesep 'lib_DiscreteDerivative.html'], '-helpbrowser')
      mask Display: disp('Discrete\nDerivative');
  FirstOrderLPF1 : Subsystem  Tag=Controls_Lib  Description=FirstOrderLowPassFilter  RTWFcnName=Derivative_1_intial  mask(First Order Low Pass Filter){}
      mask help:
      | The First Order Low Pass Filter allows signals with a frequency lower than a certain cutoff frequency (fc) to pass through the block and attenuates signals with frequencies higher than the cutoff frequency (fc or wc).
      |
      | Inputs:
      | Input        : Signal to be Filtered
      | Tau          : Filter Time Constant (1/2*pi*fc) in Seconds defined externally
      |                  by user
      | b_Reset    : Initialization flag can be used for
      |                   controlling the filter initialization
      |                   with a non-zero initial condition “ResetValue”
      |                   When b_Reset == TRUE → Out(k)=ResetValue defined externally by
      |                   user
      | ResetValue : Filter Initial Condition defined externally by user
      |
      | Output :
      | Output : Filter Output
      |
      | Notes :
      | 1. Filter time constant should be selected such that the cut-off
      |     frequency (fc)is higher than the bandwidth of the control system.
      | 2. At First sample the b_Reset should be FALSE.
      settings: RTWFileNameOpts=Use function name
      mask Help: web([fileparts(which('Lib_discrete')) filesep 'hlp' filesep 'lib_FirstOrderLPF.html'], '-helpbrowser')
      mask Display: disp('First order\nLow Pass\nFilter');
  Force2Torque : Gain  Gain=data.VEH.Re  OutDataTypeStr=Inherit: Inherit via back propagation  ParamDataTypeStr=Inherit: Same as input
  Gain : Gain  Gain=186
  Inertia : Fcn  Expr=data.VEH.Mv*(1+data.VEH.eqv_inertia)*u
  Saturation : Saturate  UpperLimit=300  LowerLimit=0
  Scope : Scope
  Scope1 : Scope
  Subsystem : Subsystem
  Sum : Sum  SaturateOnIntegerOverflow=on  InputSameDT=on  OutDataTypeStr=Inherit: Same as first input
  Torque_toforce : Gain  Gain=1/data.VEH.Re  OutDataTypeStr=Inherit: Inherit via back propagation  ParamDataTypeStr=Inherit: Same as input
  acceleration : Gain  Gain=1/data.VEH.Mv  OutDataTypeStr=Inherit: Inherit via back propagation  ParamDataTypeStr=Inherit: Same as input
  kph2ms : Gain  Gain=1/3.6  OutDataTypeStr=Inherit: Inherit via back propagation  ParamDataTypeStr=Inherit: Same as input
  m/sec2kph : Gain  Gain=3.6  OutDataTypeStr=Inherit: Inherit via back propagation  ParamDataTypeStr=Inherit: Same as input
  v_vehEstim : Outport  Tag=Controls_Lib  Description=Out  InitialOutput=0
  F_load : Outport  Tag=Controls_Lib  Description=Out  Port=2  InitialOutput=0
  dv_veh : Outport  Tag=Controls_Lib  Description=Out  Port=3  InitialOutput=0
  wires:
  brake_Request/1 -> Abs/1
  Abs/1 -> Gain/1
  M_FD/1 -> AddSub1/2
  Sum/1 -> Force2Torque/1  "F_Load"
  Force2Torque/1 -> AddSub/1
  AddSub1/1 -> Torque_toforce/1  "M_net"
  Torque_toforce/1 -> acceleration/1  "F_net"
  acceleration/1 -> Discrete-Time Integrator/1  "acceleration"
  Discrete-Time Integrator/1 -> m/sec2kph/1
  m/sec2kph/1 -> Saturation/1
  kph2ms/1 -> Inertia/1
  FirstOrderDerivative1/1(Output) -> FirstOrderLPF1/1(Input)
  Constant3/1 -> FirstOrderLPF1/2(Tau)
  Constant4/1 -> FirstOrderLPF1/3(b_Reset)
  Constant5/1 -> FirstOrderLPF1/4(ResetValue)
  [v_veh] -> FirstOrderDerivative1/1(Input)
  FirstOrderLPF1/1(Output) -> Scope1/1, dv_veh/1, [dv_veh]  "dv_veh"
  [dv_veh] -> kph2ms/1
  AddSub/1 -> AddSub1/1  "M_load"
  Gain/1 -> AddSub/2
  Inertia/1 -> Sum/2
  Saturation/1 -> Scope/1, v_vehEstim/1
  v_veh/1 -> [v_veh], Subsystem/1(v_veh)
  Subsystem/1(F_load) -> F_load/1, Sum/1

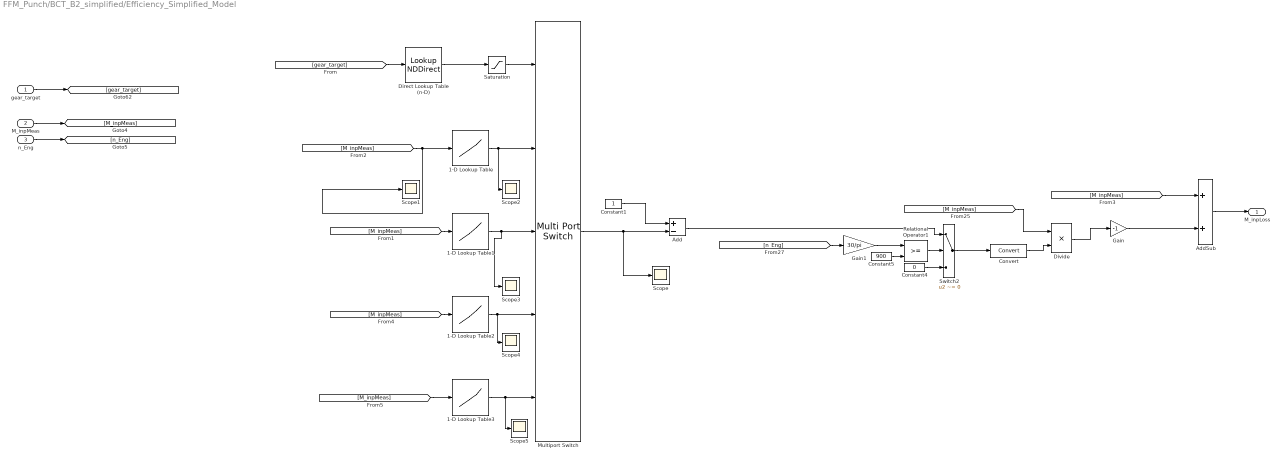
== system FFM_Punch/BCT_B2_simplified/Efficiency_Simplified_Model ==
  gear_target : Inport
  M_inpMeas : Inport  Port=2
  n_Eng : Inport  Port=3
  1-D Lookup Table : Lookup_n-D  NumberOfTableDimensions=1  BreakpointsForDimension1=data.DCT.eff_LDS012345.M_inp  Table=data.DCT.eff_LDS012345.table  InternalRulePriority=Speed  RndMeth=Simplest  InputSameDT=on
  1-D Lookup Table1 : Lookup_n-D  NumberOfTableDimensions=1  BreakpointsForDimension1=data.DCT.eff_LDS9_brake.M_inp  Table=data.DCT.eff_LDS9_brake.table  InternalRulePriority=Speed  RndMeth=Simplest  InputSameDT=on
  1-D Lookup Table2 : Lookup_n-D  NumberOfTableDimensions=1  BreakpointsForDimension1=data.DCT.eff_LDS11.M_inp  Table=data.DCT.eff_LDS11.table  InternalRulePriority=Speed  RndMeth=Simplest  InputSameDT=on
  1-D Lookup Table3 : Lookup_n-D  NumberOfTableDimensions=1  BreakpointsForDimension1=data.DCT.eff_LDS13.M_inp  Table=data.DCT.eff_LDS13.table  InternalRulePriority=Speed  RndMeth=Simplest  InputSameDT=on
  Add : Sum  Inputs=+-
  AddSub : Sum  Tag=Controls_Lib  Description=AddSub  CollapseDim=CollapseDim  AccumDataTypeStr=single  OutMin=OutMin  OutMax=OutMax  OutDataTypeStr=single  RndMeth=Nearest  SampleTime=SampleTime  InputSameDT=on  mask(AddSub){IconShape=rectangular, Inputs=++, CollapseMode=All dimensions, CollapseDim=1, SampleTime=-1, InputSameDT=on, AccumDataTypeStr=single, OutMin=[], OutMax=[], OutDataTypeStr=single, LockScale=off, RndMeth=Nearest, SaturateOnIntegerOverflow=off}
      mask prompts: IconShape "Icon shape:"; Inputs "List of signs:"; CollapseMode "Sum over:"; CollapseDim "Dimension:"; SampleTime "Sample time (-1 for inherited):"; InputSameDT "Require all inputs to have the same data type"; AccumDataTypeStr "Accumulator data type:"; OutMin "Output minimum:"; OutMax "Output maximum:"; OutDataTypeStr "Output data type:"; LockScale "Lock data type settings against changes by the fixed-point tools"; RndMeth "Integer rounding mode:"; SaturateOnIntegerOverflow "Saturate on integer overflow"
      mask help:
      | Add or subtract inputs.  Specify one of the following:
      | a) string containing + or - for each input port, | for spacer between ports (e.g. ++|-|++)
      | b) scalar, >= 1, specifies the number of input ports to be summed.
      | When there is only one input port, add or subtract elements over all dimensions or one specified dimension
      mask Help: web([fileparts(which('Lib_built')) filesep 'hlp' filesep 'lib_AddSub' '.html'], '-helpbrowser')
      mask TypeOptions IconShape: IconShape
      mask TypeOptions Inputs: Inputs
      mask TypeOptions CollapseMode: CollapseMode
      mask TypeOptions CollapseDim: CollapseDim
      mask TypeOptions SampleTime: SampleTime
      mask TypeOptions InputSameDT: InputSameDT
      mask TypeOptions AccumDataTypeStr: AccumDataTypeStr
      mask TypeOptions OutMin: OutMin
      mask TypeOptions OutMax: OutMax
      mask TypeOptions OutDataTypeStr: OutDataTypeStr
      mask TypeOptions LockScale: LockScale
      mask TypeOptions RndMeth: RndMeth
      mask TypeOptions SaturateOnIntegerOverflow: SaturateOnIntegerOverflow
  Constant1 : Constant  OutDataTypeStr=single
  Constant4 : Constant  Value=0  OutDataTypeStr=Inherit: Inherit via back propagation  SampleTime=-1
  Constant5 : Constant  Value=900  OutDataTypeStr=Inherit: Inherit via back propagation  SampleTime=-1
  Convert : DataTypeConversion  Tag=Controls_Lib  Description=Convert  OutMin=OutMin  OutMax=OutMax  RndMeth=Round  SampleTime=SampleTime  SaturateOnIntegerOverflow=on  mask(Datatype conversion){ConvertRealWorld=Real World Value (RWV), SampleTime=-1, OutMin=[], OutMax=[], OutDataTypeStr=Inherit: Inherit via back propagation, LockScale=off, RndMeth=Round, SaturateOnIntegerOverflow=on}
      mask prompts: ConvertRealWorld "Input and output to have equal:"; SampleTime "Sample time (-1 for inherited):"; OutMin "Output minimum:"; OutMax "Output maximum:"; OutDataTypeStr "Output data type:"; LockScale "Lock output data type setting against changes by the fixed-point tools"; RndMeth "Integer rounding mode:"; SaturateOnIntegerOverflow "Saturate on integer overflow"
      mask help: Convert the input to the data type and scaling of the output.
      mask Help: web([fileparts(which('Lib_built')) filesep 'hlp' filesep 'lib_DataTypeConv' '.html'], '-helpbrowser')
      mask TypeOptions ConvertRealWorld: ConvertRealWorld
      mask TypeOptions SampleTime: SampleTime
      mask TypeOptions OutMin: OutMin
      mask TypeOptions OutMax: OutMax
      mask TypeOptions OutDataTypeStr: OutDataTypeStr
      mask TypeOptions LockScale: LockScale
      mask TypeOptions RndMeth: RndMeth
      mask TypeOptions SaturateOnIntegerOverflow: SaturateOnIntegerOverflow
  Direct Lookup Table (n-D) : LookupNDDirect  NumberOfTableDimensions=1  Table=|  DiagnosticForOutOfRangeInput=None  TableDataTypeStr=single
      | [3 3 5 9 11 11 13 13
      | ]
  Divide : Product  Inputs=**
  Gain : Gain  Gain=-1
  Gain1 : Gain  Gain=30/pi
  Multiport Switch : MultiPortSwitch  DataPortOrder=Specify indices  DataPortIndices={[0,1,2,3,4,5],9,11,13}
  Relational Operator1 : RelationalOperator  OutDataTypeStr=boolean  RndMeth=Nearest  InputSameDT=on
  Saturation : Saturate  UpperLimit=13  LowerLimit=0
  Scope{,1..5} (6 alike) : Scope
  Switch2 : Switch  Criteria=u2 ~= 0  OutDataTypeStr=Inherit: Inherit via back propagation  RndMeth=Zero  SaturateOnIntegerOverflow=on  InputSameDT=on
      settings: AttributesFormatString=Criteria : %<Criteria>
  M_inpLoss : Outport
  wires:
  Saturation/1 -> Multiport Switch/1
  Direct Lookup Table (n-D)/1 -> Saturation/1
  gear_target/1 -> [gear_target]
  M_inpMeas/1 -> [M_inpMeas]
  n_Eng/1 -> [n_Eng]
  [M_inpMeas] -> Scope1/1, 1-D Lookup Table/1
  Constant1/1 -> Add/1
  Multiport Switch/1 -> Scope/1, Add/2
  [M_inpMeas] -> Divide/1
  Constant5/1 -> Relational Operator1/2
  Relational Operator1/1 -> Switch2/2
  Constant4/1 -> Switch2/3
  Switch2/1 -> Convert/1
  Add/1 -> Switch2/1
  [n_Eng] -> Gain1/1
  Gain1/1 -> Relational Operator1/1
  [gear_target] -> Direct Lookup Table (n-D)/1
  Gain/1 -> AddSub/2
  Divide/1 -> Gain/1
  [M_inpMeas] -> AddSub/1
  AddSub/1 -> M_inpLoss/1
  Convert/1 -> Divide/2
  1-D Lookup Table/1 -> Scope2/1, Multiport Switch/2
  [M_inpMeas] -> 1-D Lookup Table1/1
  [M_inpMeas] -> 1-D Lookup Table2/1
  [M_inpMeas] -> 1-D Lookup Table3/1
  1-D Lookup Table3/1 -> Scope5/1, Multiport Switch/5
  1-D Lookup Table1/1 -> Scope3/1, Multiport Switch/3
  1-D Lookup Table2/1 -> Scope4/1, Multiport Switch/4
